simulink model "IEEE14_case"  (R2024b)
settings: Solver=FixedStepAuto  StartTime=0  StopTime=2  FixedStep=1e-7  RelTol=1e-3
values from neighbouring files (symbols this model uses):
  GFL_15_Bva = 0.009    [IEEE14_parameters.m]
  GFL_15_C_bus_pu = 7.179419    [IEEE14_parameters.m]
  GFL_15_f0 = 60    [IEEE14_parameters.m]
  GFL_15_I_id = 691.26967    [IEEE14_parameters.m]
  GFL_15_I_iq = 691.26967    [IEEE14_parameters.m]
  GFL_15_I_od = 45.2207    [IEEE14_parameters.m]
  GFL_15_I_oq = 45.2207    [IEEE14_parameters.m]
  GFL_15_I_pll = 0.78    [IEEE14_parameters.m]
  GFL_15_Kdi = 0.09    [IEEE14_parameters.m]
  GFL_15_Kdo = 0.9    [IEEE14_parameters.m]
  GFL_15_Kqi = 0.09    [IEEE14_parameters.m]
  GFL_15_Kqo = 0.9    [IEEE14_parameters.m]
  GFL_15_Lg_pu = 0.631447    [IEEE14_parameters.m]
  GFL_15_mode = 1    [IEEE14_parameters.m]
  GFL_15_P_id = 3.7166    [IEEE14_parameters.m]
  GFL_15_P_iq = 3.7166    [IEEE14_parameters.m]
  GFL_15_P_od = 0.4798    [IEEE14_parameters.m]
  GFL_15_P_oq = 0.4798    [IEEE14_parameters.m]
  GFL_15_P_pll = 290.42    [IEEE14_parameters.m]
  GFL_15_Qe_ref = 0.2    [IEEE14_parameters.m]
  GFL_15_Rg_pu = 0.024016    [IEEE14_parameters.m]
  GFL_15_Sbase = 1.000000e+4    (= 10000)    [IEEE14_parameters.m]
  GFL_15_Tdi = 0.01    [IEEE14_parameters.m]
  GFL_15_Tdo = 0.2    [IEEE14_parameters.m]
  GFL_15_Tqi = 0.01    [IEEE14_parameters.m]
  GFL_15_Tqo = 0.2    [IEEE14_parameters.m]
  GFL_15_Vbase = 380    [IEEE14_parameters.m]
  GFL_15_Vdc_ref = 1.011475    [IEEE14_parameters.m]
  GFL_15_Vdcbase = 700    [IEEE14_parameters.m]
  GFL_15_vq_ref = 0    [IEEE14_parameters.m]
  GFL_16_Bva = 0.002    [IEEE14_parameters.m]
  GFL_16_C_bus_pu = 7.179419    [IEEE14_parameters.m]
  GFL_16_f0 = 60    [IEEE14_parameters.m]
  GFL_16_I_id = 691.26967    [IEEE14_parameters.m]
  GFL_16_I_iq = 691.26967    [IEEE14_parameters.m]
  GFL_16_I_od = 45.2207    [IEEE14_parameters.m]
  GFL_16_I_oq = 45.2207    [IEEE14_parameters.m]
  GFL_16_I_pll = 0.78    [IEEE14_parameters.m]
  GFL_16_Kdi = 0.05    [IEEE14_parameters.m]
  GFL_16_Kdo = 0.5    [IEEE14_parameters.m]
  GFL_16_Kqi = 0.05    [IEEE14_parameters.m]
  GFL_16_Kqo = 0.5    [IEEE14_parameters.m]
  GFL_16_Lg_pu = 0.631447    [IEEE14_parameters.m]
  GFL_16_mode = 1    [IEEE14_parameters.m]
  GFL_16_P_id = 3.7166    [IEEE14_parameters.m]
  GFL_16_P_iq = 3.7166    [IEEE14_parameters.m]
  GFL_16_P_od = 0.4798    [IEEE14_parameters.m]
  GFL_16_P_oq = 0.4798    [IEEE14_parameters.m]
  GFL_16_P_pll = 290.42    [IEEE14_parameters.m]
  GFL_16_Qe_ref = 0.2    [IEEE14_parameters.m]
  GFL_16_Rg_pu = 0.024016    [IEEE14_parameters.m]
  GFL_16_Sbase = 1.000000e+4    (= 10000)    [IEEE14_parameters.m]
  GFL_16_Tdi = 0.01    [IEEE14_parameters.m]
  GFL_16_Tdo = 0.2    [IEEE14_parameters.m]
  GFL_16_Tqi = 0.01    [IEEE14_parameters.m]
  GFL_16_Tqo = 0.2    [IEEE14_parameters.m]
  GFL_16_Vbase = 380    [IEEE14_parameters.m]
  GFL_16_Vdc_ref = 1.01144    [IEEE14_parameters.m]
  GFL_16_Vdcbase = 700    [IEEE14_parameters.m]
  GFL_16_vq_ref = 0    [IEEE14_parameters.m]
  GFL_17_Bva = 0.002    [IEEE14_parameters.m]
  GFL_17_C_bus_pu = 7.179419    [IEEE14_parameters.m]
  GFL_17_f0 = 60    [IEEE14_parameters.m]
  GFL_17_I_id = 691.26967    [IEEE14_parameters.m]
  GFL_17_I_iq = 691.26967    [IEEE14_parameters.m]
  GFL_17_I_od = 45.2207    [IEEE14_parameters.m]
  GFL_17_I_oq = 45.2207    [IEEE14_parameters.m]
  GFL_17_I_pll = 0.78    [IEEE14_parameters.m]
  GFL_17_Kdi = 0.05    [IEEE14_parameters.m]
  GFL_17_Kdo = 0.5    [IEEE14_parameters.m]
  GFL_17_Kqi = 0.05    [IEEE14_parameters.m]
  GFL_17_Kqo = 0.5    [IEEE14_parameters.m]
  GFL_17_Lg_pu = 0.631447    [IEEE14_parameters.m]
  GFL_17_mode = 1    [IEEE14_parameters.m]
  GFL_17_P_id = 3.7166    [IEEE14_parameters.m]
  GFL_17_P_iq = 3.7166    [IEEE14_parameters.m]
  GFL_17_P_od = 0.4798    [IEEE14_parameters.m]
  GFL_17_P_oq = 0.4798    [IEEE14_parameters.m]
  GFL_17_P_pll = 290.42    [IEEE14_parameters.m]
  GFL_17_Qe_ref = 0.2    [IEEE14_parameters.m]
  GFL_17_Rg_pu = 0.024016    [IEEE14_parameters.m]
  GFL_17_Sbase = 1.000000e+4    (= 10000)    [IEEE14_parameters.m]
  GFL_17_Tdi = 0.01    [IEEE14_parameters.m]
  GFL_17_Tdo = 0.2    [IEEE14_parameters.m]
  GFL_17_Tqi = 0.01    [IEEE14_parameters.m]
  GFL_17_Tqo = 0.2    [IEEE14_parameters.m]
  GFL_17_Vbase = 380    [IEEE14_parameters.m]
  GFL_17_Vdc_ref = 1.011632    [IEEE14_parameters.m]
  GFL_17_Vdcbase = 700    [IEEE14_parameters.m]
  GFL_17_vq_ref = 0    [IEEE14_parameters.m]
  GFL_18_Bva = 0.002    [IEEE14_parameters.m]
  GFL_18_C_bus_pu = 7.179419    [IEEE14_parameters.m]
  GFL_18_f0 = 60    [IEEE14_parameters.m]
  GFL_18_I_id = 691.26967    [IEEE14_parameters.m]
  GFL_18_I_iq = 691.26967    [IEEE14_parameters.m]
  GFL_18_I_od = 45.2207    [IEEE14_parameters.m]
  GFL_18_I_oq = 45.2207    [IEEE14_parameters.m]
  GFL_18_I_pll = 0.78    [IEEE14_parameters.m]
  GFL_18_Kdi = 0.05    [IEEE14_parameters.m]
  GFL_18_Kdo = 0.5    [IEEE14_parameters.m]
  GFL_18_Kqi = 0.05    [IEEE14_parameters.m]
  GFL_18_Kqo = 0.5    [IEEE14_parameters.m]
  GFL_18_Lg_pu = 0.631447    [IEEE14_parameters.m]
  GFL_18_mode = 1    [IEEE14_parameters.m]
  GFL_18_P_id = 3.7166    [IEEE14_parameters.m]
  GFL_18_P_iq = 3.7166    [IEEE14_parameters.m]
  GFL_18_P_od = 0.4798    [IEEE14_parameters.m]
  GFL_18_P_oq = 0.4798    [IEEE14_parameters.m]
  GFL_18_P_pll = 290.42    [IEEE14_parameters.m]
  GFL_18_Qe_ref = 0.2    [IEEE14_parameters.m]
  GFL_18_Rg_pu = 0.024016    [IEEE14_parameters.m]
  GFL_18_Sbase = 1.000000e+4    (= 10000)    [IEEE14_parameters.m]
  GFL_18_Tdi = 0.01    [IEEE14_parameters.m]
  GFL_18_Tdo = 0.2    [IEEE14_parameters.m]
  GFL_18_Tqi = 0.01    [IEEE14_parameters.m]
  GFL_18_Tqo = 0.2    [IEEE14_parameters.m]
  GFL_18_Vbase = 380    [IEEE14_parameters.m]
  GFL_18_Vdc_ref = 1.011572    [IEEE14_parameters.m]
  GFL_18_Vdcbase = 700    [IEEE14_parameters.m]
  GFL_18_vq_ref = 0    [IEEE14_parameters.m]
  ... (+180 more)
(part 20 of 25)

== system IEEE14_case/SG_D_3/d_psi_fd_SG_D_3_block ==
  note: d_psi_fd_SG_D_3 in case14gfl
      | $-\frac{\psi _{\mathrm{fd},\mathrm{SG},D,3}-E_{\mathrm{fd},\mathrm{SG},D,3}+\left(x_{d}-x_{\mathrm{dd}}\right)\,\left(\frac{\frac{\psi _{\mathrm{1d},\mathrm{SG},D,3}\,\left(x_{\mathrm{dd}}-x_{\mathrm{ddd}}\right)}{x_{\mathrm{dd}}-x_{l}}-\psi _{d,\mathrm{SG},D,3}+\frac{\psi _{\mathrm{fd},\mathrm{SG},D,3}\,\left(x_{\mathrm{ddd}}-x_{l}\right)}{x_{\mathrm{dd}}-x_{l}}}{x_{\mathrm{ddd}}}-\frac{\left(x_{\mathrm{dd}}-x_{\mathrm{ddd}}\right)\,\left(\psi _{\mathrm{1d},\mathrm{SG},D,3}-\psi _{\mathrm{fd},\mathrm{SG},D,3}+\frac{\left(x_{\mathrm{dd}}-x_{l}\right)\,\left(\frac{\psi _{\mathrm{1d},\mathrm{SG},D,3}\,\left(x_{\mathrm{dd}}-x_{\mathrm{ddd}}\right)}{x_{\mathrm{dd}}-x_{l}}-\psi _{d,\mathrm{SG},D,3}+\frac{\psi _{\mathrm{fd},\mathrm{SG},D,3}\,\left(x_{\mathrm{ddd}}-x_{l}\right)}{x_{\mathrm{dd}}-x_{l}}\right)}{x_{\mathrm{ddd}}}\right)}{{\left(x_{\mathrm{dd}}-x_{l}\right)}^2}\right)}{T_{\mathrm{dd}}}$
      | Automatically generated on 2025-10-09 21:31:58 .
  State_E_fd_SG_D_3_d78e2 : Inport
  State_psi_fd_SG_D_3_1ca94 : Inport  Port=2
  State_psi_1d_SG_D_3_100d0 : Inport  Port=3
  State_psi_fd_SG_D_3_1fedc : Inport  Port=4
  State_psi_1d_SG_D_3_43bed : Inport  Port=5
  State_psi_d_SG_D_3_d3054 : Inport  Port=6
  State_psi_fd_SG_D_3_13cfd : Inport  Port=7
  State_psi_1d_SG_D_3_3ce6e : Inport  Port=8
  State_psi_d_SG_D_3_4847b : Inport  Port=9
  State_psi_fd_SG_D_3_01d8a : Inport  Port=10
  Add_80d2e : Sum
  Add_c54d7 : Sum
  Constant_-1_b236f : Constant  Value=-1
  Constant_-1_bec81 : Constant  Value=-1
  Constant_-1_d1f6f : Constant  Value=-1
  Constant_2.0_9c0bc : Constant  Value=2.0
  Constant_T_dd_bb507 : Constant  Value=T_dd
  Constant_x_d_3177e : Constant  Value=x_d
  Constant_x_dd_197e1 : Constant  Value=x_dd
  Constant_x_dd_2f9f2 : Constant  Value=x_dd
  Constant_x_dd_2fa42 : Constant  Value=x_dd
  Constant_x_dd_34495 : Constant  Value=x_dd
  Constant_x_dd_5dc80 : Constant  Value=x_dd
  Constant_x_dd_8bf3f : Constant  Value=x_dd
  Constant_x_dd_a9902 : Constant  Value=x_dd
  Constant_x_dd_c1224 : Constant  Value=x_dd
  Constant_x_dd_d2500 : Constant  Value=x_dd
  Constant_x_dd_f7ff0 : Constant  Value=x_dd
  Constant_x_ddd_238d1 : Constant  Value=x_ddd
  Constant_x_ddd_5390a : Constant  Value=x_ddd
  Constant_x_ddd_826ba : Constant  Value=x_ddd
  Constant_x_ddd_b0317 : Constant  Value=x_ddd
  Constant_x_ddd_b32cc : Constant  Value=x_ddd
  Constant_x_ddd_c2563 : Constant  Value=x_ddd
  Constant_x_ddd_db75c : Constant  Value=x_ddd
  Constant_x_l_1a217 : Constant  Value=x_l
  Constant_x_l_22cc2 : Constant  Value=x_l
  Constant_x_l_244ba : Constant  Value=x_l
  Constant_x_l_454cb : Constant  Value=x_l
  Constant_x_l_5313e : Constant  Value=x_l
  Constant_x_l_96c37 : Constant  Value=x_l
  Constant_x_l_de542 : Constant  Value=x_l
  Constant_x_l_e5b53 : Constant  Value=x_l
  Divide_0852c : Product  Inputs=*/
  Divide_3c28e : Product  Inputs=*/
  Divide_3c654 : Product  Inputs=*/
  Divide_63bfa : Product  Inputs=*/
  Divide_677e2 : Product  Inputs=*/
  Divide_9dd51 : Product  Inputs=*/
  Divide_a3d2d : Product  Inputs=*/
  Divide_c5de7 : Product  Inputs=*/
  Power_b9f7a : Math  Operator=pow
  Product_029d7 : Product
  Product_1e69a : Product
  Product_2ea94 : Product
  Product_9be52 : Product
  Product_a7353 : Product
  Product_b7520 : Product
  Product_b932f : Product
  Product_c4689 : Product
  Product_d1d0a : Product
  Product_dc8c2 : Product
  Subtract_0348b : Sum  Inputs=+-
  Subtract_12722 : Sum  Inputs=+-
  Subtract_267a6 : Sum  Inputs=+-
  Subtract_26a75 : Sum  Inputs=+-
  Subtract_468ee : Sum  Inputs=+-
  Subtract_48e53 : Sum  Inputs=+-
  Subtract_4fd9e : Sum  Inputs=+-
  Subtract_5d9ec : Sum  Inputs=+-
  Subtract_60539 : Sum  Inputs=+-
  Subtract_67c8f : Sum  Inputs=+-
  Subtract_905f1 : Sum  Inputs=+-
  Subtract_a0641 : Sum  Inputs=+-
  Subtract_a2941 : Sum  Inputs=+-
  Subtract_a6db3 : Sum  Inputs=+-
  Subtract_b8cef : Sum  Inputs=+-
  Subtract_c861a : Sum  Inputs=+-
  Subtract_db6b7 : Sum  Inputs=+-
  Subtract_ddf1e : Sum  Inputs=+-
  Subtract_df264 : Sum  Inputs=+-
  Blockout_d_psi_fd_SG_D_3_d4122 : Outport
  wires:
  Product_a7353/1 -> Divide_3c28e/1
  Constant_-1_b236f/1 -> Product_c4689/1
  Subtract_468ee/1 -> Product_2ea94/2
  State_psi_1d_SG_D_3_43bed/1 -> Product_c4689/2
  Constant_x_l_5313e/1 -> Subtract_a2941/2
  Constant_x_dd_5dc80/1 -> Subtract_468ee/1
  Constant_x_ddd_b32cc/1 -> Subtract_468ee/2
  Product_c4689/1 -> Product_2ea94/1
  Constant_x_dd_a9902/1 -> Subtract_db6b7/1
  Constant_x_l_454cb/1 -> Subtract_db6b7/2
  Constant_x_ddd_5390a/1 -> Subtract_5d9ec/2
  Constant_x_ddd_b0317/1 -> Subtract_26a75/1
  Constant_x_l_244ba/1 -> Subtract_26a75/2
  Product_b932f/1 -> Product_d1d0a/1
  Product_2ea94/1 -> Divide_3c654/1
  Subtract_db6b7/1 -> Divide_3c654/2
  State_psi_fd_SG_D_3_13cfd/1 -> Product_029d7/1
  Constant_x_ddd_db75c/1 -> Subtract_a2941/1
  Subtract_26a75/1 -> Product_029d7/2
  Constant_x_dd_8bf3f/1 -> Subtract_c861a/1
  Constant_-1_bec81/1 -> Product_b932f/1
  Constant_x_l_e5b53/1 -> Subtract_c861a/2
  Product_d1d0a/1 -> Divide_677e2/1
  Divide_3c654/1 -> Add_80d2e/1
  Product_b7520/1 -> Divide_0852c/1
  State_psi_d_SG_D_3_d3054/1 -> Add_80d2e/2
  State_psi_fd_SG_D_3_01d8a/1 -> Product_b7520/1
  Product_029d7/1 -> Divide_a3d2d/1
  Constant_x_dd_197e1/1 -> Subtract_905f1/1
  Subtract_c861a/1 -> Divide_a3d2d/2
  Constant_x_l_96c37/1 -> Subtract_ddf1e/2
  Constant_x_dd_d2500/1 -> Subtract_b8cef/1
  Subtract_267a6/1 -> Product_dc8c2/2
  Constant_x_l_1a217/1 -> Subtract_b8cef/2
  Divide_677e2/1 -> Add_c54d7/1
  Constant_x_ddd_826ba/1 -> Divide_3c28e/2
  Add_80d2e/1 -> Subtract_12722/1
  Divide_a3d2d/1 -> Subtract_12722/2
  State_psi_1d_SG_D_3_3ce6e/1 -> Product_b932f/2
  Constant_x_l_de542/1 -> Subtract_905f1/2
  Constant_x_dd_2f9f2/1 -> Subtract_5d9ec/1
  Subtract_b8cef/1 -> Product_a7353/1
  Add_c54d7/1 -> Subtract_67c8f/1
  Subtract_12722/1 -> Product_a7353/2
  Subtract_5d9ec/1 -> Product_d1d0a/2
  Constant_x_dd_f7ff0/1 -> Subtract_60539/1
  Constant_x_l_22cc2/1 -> Subtract_60539/2
  Subtract_a2941/1 -> Product_b7520/2
  Constant_x_dd_34495/1 -> Subtract_267a6/1
  Constant_x_ddd_238d1/1 -> Subtract_267a6/2
  Product_dc8c2/1 -> Product_9be52/1
  State_psi_1d_SG_D_3_100d0/1 -> Subtract_df264/1
  Subtract_60539/1 -> Divide_677e2/2
  State_psi_fd_SG_D_3_1fedc/1 -> Subtract_df264/2
  Constant_-1_d1f6f/1 -> Product_dc8c2/1
  Subtract_df264/1 -> Subtract_a0641/1
  Divide_3c28e/1 -> Subtract_a0641/2
  Constant_x_dd_c1224/1 -> Subtract_ddf1e/1
  Divide_0852c/1 -> Subtract_67c8f/2
  State_psi_d_SG_D_3_4847b/1 -> Add_c54d7/2
  Subtract_905f1/1 -> Divide_0852c/2
  Subtract_a0641/1 -> Product_9be52/2
  Subtract_ddf1e/1 -> Power_b9f7a/1
  Constant_2.0_9c0bc/1 -> Power_b9f7a/2
  Product_9be52/1 -> Divide_c5de7/1
  Subtract_48e53/1 -> Product_1e69a/2
  Power_b9f7a/1 -> Divide_c5de7/2
  Subtract_67c8f/1 -> Divide_63bfa/1
  Constant_x_ddd_c2563/1 -> Divide_63bfa/2
  Constant_x_d_3177e/1 -> Subtract_0348b/1
  Constant_x_dd_2fa42/1 -> Subtract_0348b/2
  Divide_c5de7/1 -> Subtract_48e53/1
  Divide_63bfa/1 -> Subtract_48e53/2
  State_E_fd_SG_D_3_d78e2/1 -> Subtract_a6db3/1
  State_psi_fd_SG_D_3_1ca94/1 -> Subtract_a6db3/2
  Subtract_0348b/1 -> Product_1e69a/1
  Subtract_a6db3/1 -> Subtract_4fd9e/1
  Product_1e69a/1 -> Subtract_4fd9e/2
  Subtract_4fd9e/1 -> Divide_9dd51/1
  Constant_T_dd_bb507/1 -> Divide_9dd51/2
  Divide_9dd51/1 -> Blockout_d_psi_fd_SG_D_3_d4122/1

== system IEEE14_case/SG_D_3/d_psi_gq_SG_D_3_block ==
  note: d_psi_gq_SG_D_3 in case14gfl
      | $-\frac{\psi _{\mathrm{gq},\mathrm{SG},D,3}+\left(x_{q}-x_{\mathrm{qd}}\right)\,\left(\frac{\psi _{q,\mathrm{SG},D,3}+\frac{\psi _{\mathrm{gq},\mathrm{SG},D,3}\,\left(x_{l}-x_{\mathrm{qdd}}\right)}{x_{l}-x_{\mathrm{qd}}}+\frac{\psi _{\mathrm{kq},\mathrm{SG},D,3}\,\left(x_{\mathrm{qd}}-x_{\mathrm{qdd}}\right)}{x_{l}-x_{\mathrm{qd}}}}{x_{\mathrm{qdd}}}+\frac{\left(x_{\mathrm{qd}}-x_{\mathrm{qdd}}\right)\,\left(\psi _{\mathrm{gq},\mathrm{SG},D,3}+\psi _{\mathrm{kq},\mathrm{SG},D,3}+\frac{\left(x_{l}-x_{\mathrm{qd}}\right)\,\left(\psi _{q,\mathrm{SG},D,3}+\frac{\psi _{\mathrm{gq},\mathrm{SG},D,3}\,\left(x_{l}-x_{\mathrm{qdd}}\right)}{x_{l}-x_{\mathrm{qd}}}+\frac{\psi _{\mathrm{kq},\mathrm{SG},D,3}\,\left(x_{\mathrm{qd}}-x_{\mathrm{qdd}}\right)}{x_{l}-x_{\mathrm{qd}}}\right)}{x_{\mathrm{qdd}}}\right)}{{\left(x_{l}-x_{\mathrm{qd}}\right)}^2}\right)}{T_{\mathrm{qd}}}$
      | Automatically generated on 2025-10-09 21:32:05 .
  State_psi_gq_SG_D_3_61d89 : Inport
  State_psi_gq_SG_D_3_d2fbb : Inport  Port=2
  State_psi_kq_SG_D_3_dfb0b : Inport  Port=3
  State_psi_gq_SG_D_3_45fb4 : Inport  Port=4
  State_psi_kq_SG_D_3_5ef0d : Inport  Port=5
  State_psi_q_SG_D_3_2ea70 : Inport  Port=6
  State_psi_gq_SG_D_3_a842f : Inport  Port=7
  State_psi_kq_SG_D_3_da800 : Inport  Port=8
  State_psi_q_SG_D_3_77fff : Inport  Port=9
  Add_74d59 : Sum
  Add_80cf5 : Sum
  Add_88f67 : Sum
  Add_8b6d3 : Sum
  Add_96fed : Sum
  Add_a22ad : Sum
  Add_a2434 : Sum
  Add_a3f81 : Sum
  Add_ba19f : Sum
  Add_e5f57 : Sum
  Add_f7575 : Sum
  Add_fd6a4 : Sum
  Constant_-1_073cf : Constant  Value=-1
  Constant_-1_20b8e : Constant  Value=-1
  Constant_-1_2bb06 : Constant  Value=-1
  Constant_-1_56ef8 : Constant  Value=-1
  Constant_-1_8bd02 : Constant  Value=-1
  Constant_-1_b65c8 : Constant  Value=-1
  Constant_-1_d4353 : Constant  Value=-1
  Constant_-1_de30b : Constant  Value=-1
  Constant_-1_e0e58 : Constant  Value=-1
  Constant_-1_e21ce : Constant  Value=-1
  Constant_2.0_954e6 : Constant  Value=2.0
  Constant_T_qd_c4423 : Constant  Value=T_qd
  Constant_x_l_1b9e5 : Constant  Value=x_l
  Constant_x_l_37ca8 : Constant  Value=x_l
  Constant_x_l_61450 : Constant  Value=x_l
  Constant_x_l_620cb : Constant  Value=x_l
  Constant_x_l_67d60 : Constant  Value=x_l
  Constant_x_l_adcf0 : Constant  Value=x_l
  Constant_x_l_bd098 : Constant  Value=x_l
  Constant_x_l_e870d : Constant  Value=x_l
  Constant_x_q_9ac0a : Constant  Value=x_q
  Constant_x_qd_04582 : Constant  Value=x_qd
  Constant_x_qd_08b35 : Constant  Value=x_qd
  Constant_x_qd_108e4 : Constant  Value=x_qd
  Constant_x_qd_11bce : Constant  Value=x_qd
  Constant_x_qd_321d1 : Constant  Value=x_qd
  Constant_x_qd_56097 : Constant  Value=x_qd
  Constant_x_qd_8aa9c : Constant  Value=x_qd
  Constant_x_qd_bf5b6 : Constant  Value=x_qd
  Constant_x_qd_d07df : Constant  Value=x_qd
  Constant_x_qd_f5adf : Constant  Value=x_qd
  Constant_x_qdd_27f87 : Constant  Value=x_qdd
  Constant_x_qdd_38975 : Constant  Value=x_qdd
  Constant_x_qdd_467dc : Constant  Value=x_qdd
  Constant_x_qdd_9fc2a : Constant  Value=x_qdd
  Constant_x_qdd_b0870 : Constant  Value=x_qdd
  Constant_x_qdd_b80c6 : Constant  Value=x_qdd
  Constant_x_qdd_f1e40 : Constant  Value=x_qdd
  Divide_00b90 : Product  Inputs=*/
  Divide_023dc : Product  Inputs=*/
  Divide_04f18 : Product  Inputs=*/
  Divide_3584c : Product  Inputs=*/
  Divide_4654a : Product  Inputs=*/
  Divide_4d5e7 : Product  Inputs=*/
  Divide_7f03c : Product  Inputs=*/
  Divide_b9d54 : Product  Inputs=*/
  Power_20cbb : Math  Operator=pow
  Product_0547a : Product
  Product_24422 : Product
  Product_2fb4f : Product
  Product_393f7 : Product
  Product_7f4c8 : Product
  Product_85de0 : Product
  Product_8b155 : Product
  Product_9510e : Product
  Product_a76f8 : Product
  Product_a7e86 : Product
  Product_b4629 : Product
  Product_b6ffa : Product
  Product_cb497 : Product
  Product_d015c : Product
  Product_de0ec : Product
  Product_e96c0 : Product
  Product_f73f6 : Product
  Subtract_0e44b : Sum  Inputs=+-
  Subtract_4270b : Sum  Inputs=+-
  Subtract_67b07 : Sum  Inputs=+-
  Subtract_96d88 : Sum  Inputs=+-
  Subtract_b3885 : Sum  Inputs=+-
  Subtract_c23cf : Sum  Inputs=+-
  Subtract_df751 : Sum  Inputs=+-
  Subtract_dfb85 : Sum  Inputs=+-
  Blockout_d_psi_gq_SG_D_3_d5302 : Outport
  wires:
  Constant_x_l_37ca8/1 -> Product_e96c0/2
  Constant_x_qd_108e4/1 -> Subtract_dfb85/1
  Add_e5f57/1 -> Product_b4629/1
  Constant_-1_2bb06/1 -> Product_0547a/1
  Add_fd6a4/1 -> Product_8b155/2
  Constant_x_qdd_b0870/1 -> Subtract_dfb85/2
  Constant_x_qd_04582/1 -> Add_e5f57/2
  Constant_x_l_adcf0/1 -> Product_0547a/2
  Constant_x_l_620cb/1 -> Product_9510e/2
  Add_ba19f/1 -> Divide_4654a/2
  State_psi_kq_SG_D_3_dfb0b/1 -> Add_a3f81/2
  Constant_x_qdd_9fc2a/1 -> Add_fd6a4/2
  Product_0547a/1 -> Add_fd6a4/1
  Constant_x_qd_bf5b6/1 -> Add_ba19f/2
  Product_393f7/1 -> Product_f73f6/1
  Constant_-1_e0e58/1 -> Product_2fb4f/1
  Constant_-1_8bd02/1 -> Product_9510e/1
  Constant_-1_073cf/1 -> Product_85de0/1
  Constant_x_l_61450/1 -> Product_85de0/2
  Constant_-1_e21ce/1 -> Product_393f7/1
  Constant_-1_b65c8/1 -> Product_24422/1
  State_psi_gq_SG_D_3_45fb4/1 -> Product_8b155/1
  Product_2fb4f/1 -> Add_a2434/1
  Product_9510e/1 -> Add_a22ad/1
  Product_7f4c8/1 -> Add_ba19f/1
  Constant_x_qd_08b35/1 -> Add_a22ad/2
  Constant_-1_56ef8/1 -> Product_a7e86/1
  State_psi_kq_SG_D_3_5ef0d/1 -> Product_b6ffa/1
  Subtract_dfb85/1 -> Product_b6ffa/2
  Product_85de0/1 -> Add_88f67/1
  Add_a2434/1 -> Product_d015c/2
  Add_a22ad/1 -> Divide_3584c/2
  Constant_x_qd_f5adf/1 -> Add_88f67/2
  Product_8b155/1 -> Divide_3584c/1
  Constant_T_qd_c4423/1 -> Divide_023dc/2
  Product_a7e86/1 -> Add_74d59/1
  Product_b6ffa/1 -> Divide_00b90/1
  Product_a76f8/1 -> Divide_4654a/1
  Add_88f67/1 -> Divide_00b90/2
  Constant_-1_d4353/1 -> Product_cb497/1
  Constant_x_qdd_467dc/1 -> Divide_b9d54/2
  Constant_x_l_e870d/1 -> Product_cb497/2
  Divide_3584c/1 -> Subtract_df751/1
  Constant_x_qd_d07df/1 -> Subtract_c23cf/2
  Add_74d59/1 -> Divide_4d5e7/2
  Divide_00b90/1 -> Subtract_df751/2
  Constant_x_l_1b9e5/1 -> Product_2fb4f/2
  Product_cb497/1 -> Add_e5f57/1
  Constant_-1_de30b/1 -> Product_e96c0/1
  Constant_x_l_67d60/1 -> Product_a7e86/2
  Subtract_df751/1 -> Add_96fed/1
  State_psi_q_SG_D_3_2ea70/1 -> Add_96fed/2
  Constant_-1_20b8e/1 -> Product_7f4c8/1
  Constant_x_qdd_b80c6/1 -> Add_a2434/2
  Constant_x_qd_56097/1 -> Subtract_96d88/1
  Constant_x_qdd_38975/1 -> Subtract_96d88/2
  Constant_x_l_bd098/1 -> Product_7f4c8/2
  Add_96fed/1 -> Product_b4629/2
  Constant_x_qdd_27f87/1 -> Subtract_67b07/2
  State_psi_gq_SG_D_3_a842f/1 -> Product_d015c/1
  Constant_x_qd_8aa9c/1 -> Add_74d59/2
  Divide_7f03c/1 -> Subtract_b3885/1
  State_psi_kq_SG_D_3_da800/1 -> Product_a76f8/1
  Subtract_96d88/1 -> Product_a76f8/2
  Constant_x_qd_11bce/1 -> Subtract_67b07/1
  State_psi_gq_SG_D_3_d2fbb/1 -> Add_a3f81/1
  Product_b4629/1 -> Divide_b9d54/1
  Product_d015c/1 -> Divide_4d5e7/1
  Subtract_67b07/1 -> Product_393f7/2
  Add_a3f81/1 -> Subtract_0e44b/1
  Divide_b9d54/1 -> Subtract_0e44b/2
  Product_e96c0/1 -> Add_80cf5/1
  Constant_x_qd_321d1/1 -> Add_80cf5/2
  Divide_4d5e7/1 -> Subtract_4270b/1
  Divide_4654a/1 -> Subtract_4270b/2
  Subtract_0e44b/1 -> Product_f73f6/2
  Add_80cf5/1 -> Power_20cbb/1
  Constant_2.0_954e6/1 -> Power_20cbb/2
  Subtract_4270b/1 -> Add_f7575/1
  State_psi_q_SG_D_3_77fff/1 -> Add_f7575/2
  Product_f73f6/1 -> Divide_7f03c/1
  Power_20cbb/1 -> Divide_7f03c/2
  Add_f7575/1 -> Divide_04f18/1
  Constant_x_qdd_f1e40/1 -> Divide_04f18/2
  Constant_x_q_9ac0a/1 -> Subtract_c23cf/1
  Divide_04f18/1 -> Subtract_b3885/2
  State_psi_gq_SG_D_3_61d89/1 -> Product_24422/2
  Subtract_c23cf/1 -> Product_de0ec/1
  Subtract_b3885/1 -> Product_de0ec/2
  Product_24422/1 -> Add_8b6d3/1
  Product_de0ec/1 -> Add_8b6d3/2
  Add_8b6d3/1 -> Divide_023dc/1
  Divide_023dc/1 -> Blockout_d_psi_gq_SG_D_3_d5302/1

== system IEEE14_case/SG_D_3/d_psi_kq_SG_D_3_block ==
  note: d_psi_kq_SG_D_3 in case14gfl
      | $-\frac{\psi _{\mathrm{gq},\mathrm{SG},D,3}+\psi _{\mathrm{kq},\mathrm{SG},D,3}+\frac{\left(x_{l}-x_{\mathrm{qd}}\right)\,\left(\psi _{q,\mathrm{SG},D,3}+\frac{\psi _{\mathrm{gq},\mathrm{SG},D,3}\,\left(x_{l}-x_{\mathrm{qdd}}\right)}{x_{l}-x_{\mathrm{qd}}}+\frac{\psi _{\mathrm{kq},\mathrm{SG},D,3}\,\left(x_{\mathrm{qd}}-x_{\mathrm{qdd}}\right)}{x_{l}-x_{\mathrm{qd}}}\right)}{x_{\mathrm{qdd}}}}{T_{\mathrm{qdd}}}$
      | Automatically generated on 2025-10-09 21:32:08 .
  State_psi_gq_SG_D_3_5f103 : Inport
  State_psi_kq_SG_D_3_66cec : Inport  Port=2
  State_psi_gq_SG_D_3_d768f : Inport  Port=3
  State_psi_kq_SG_D_3_3bd28 : Inport  Port=4
  State_psi_q_SG_D_3_41969 : Inport  Port=5
  Add_0ddbf : Sum
  Add_1aa52 : Sum
  Add_51ab7 : Sum
  Add_8654d : Sum
  Add_a36c4 : Sum
  Add_d72a9 : Sum
  Constant_-1_02b02 : Constant  Value=-1
  Constant_-1_0d781 : Constant  Value=-1
  Constant_-1_99886 : Constant  Value=-1
  Constant_-1_d75ef : Constant  Value=-1
  Constant_-1_d97d4 : Constant  Value=-1
  Constant_T_qdd_6762e : Constant  Value=T_qdd
  Constant_x_l_0960a : Constant  Value=x_l
  Constant_x_l_772c1 : Constant  Value=x_l
  Constant_x_l_c951c : Constant  Value=x_l
  Constant_x_l_f41cc : Constant  Value=x_l
  Constant_x_qd_7ea52 : Constant  Value=x_qd
  Constant_x_qd_b6964 : Constant  Value=x_qd
  Constant_x_qd_c158b : Constant  Value=x_qd
  Constant_x_qd_d1d5f : Constant  Value=x_qd
  Constant_x_qdd_3258c : Constant  Value=x_qdd
  Constant_x_qdd_6ba2b : Constant  Value=x_qdd
  Constant_x_qdd_72f52 : Constant  Value=x_qdd
  Divide_28285 : Product  Inputs=*/
  Divide_2d6a6 : Product  Inputs=*/
  Divide_38392 : Product  Inputs=*/
  Divide_ec21f : Product  Inputs=*/
  Product_064ec : Product
  Product_0c2ce : Product
  Product_5b1b5 : Product
  Product_67d15 : Product
  Product_7b1df : Product
  Product_8a972 : Product
  Product_de990 : Product
  Product_ed944 : Product
  Subtract_516d0 : Sum  Inputs=+-
  Subtract_808b2 : Sum  Inputs=+-
  Subtract_a4f43 : Sum  Inputs=+-
  Blockout_d_psi_kq_SG_D_3_bc348 : Outport
  wires:
  State_psi_q_SG_D_3_41969/1 -> Add_1aa52/2
  Constant_-1_d75ef/1 -> Product_0c2ce/1
  Constant_-1_99886/1 -> Product_de990/1
  Constant_-1_0d781/1 -> Product_ed944/1
  Constant_x_l_0960a/1 -> Product_0c2ce/2
  Constant_x_qdd_72f52/1 -> Add_51ab7/2
  Product_8a972/1 -> Add_8654d/1
  Constant_x_l_772c1/1 -> Product_de990/2
  Constant_x_qd_c158b/1 -> Subtract_516d0/1
  Product_de990/1 -> Add_51ab7/1
  Constant_x_l_c951c/1 -> Product_5b1b5/2
  Constant_x_qdd_6ba2b/1 -> Subtract_516d0/2
  Constant_-1_d97d4/1 -> Product_8a972/1
  Constant_x_l_f41cc/1 -> Product_8a972/2
  State_psi_gq_SG_D_3_d768f/1 -> Product_67d15/1
  Add_51ab7/1 -> Product_67d15/2
  Add_1aa52/1 -> Product_7b1df/2
  Product_0c2ce/1 -> Add_d72a9/1
  Constant_x_qd_d1d5f/1 -> Add_d72a9/2
  State_psi_kq_SG_D_3_3bd28/1 -> Product_064ec/1
  Subtract_516d0/1 -> Product_064ec/2
  Add_d72a9/1 -> Divide_2d6a6/2
  Constant_x_qd_b6964/1 -> Add_8654d/2
  Product_67d15/1 -> Divide_2d6a6/1
  Product_064ec/1 -> Divide_ec21f/1
  Add_8654d/1 -> Divide_ec21f/2
  Constant_-1_02b02/1 -> Product_5b1b5/1
  Divide_2d6a6/1 -> Subtract_a4f43/1
  Add_a36c4/1 -> Divide_38392/1
  Divide_ec21f/1 -> Subtract_a4f43/2
  Divide_38392/1 -> Blockout_d_psi_kq_SG_D_3_bc348/1
  Product_5b1b5/1 -> Add_0ddbf/1
  Constant_x_qd_7ea52/1 -> Add_0ddbf/2
  Subtract_a4f43/1 -> Add_1aa52/1
  State_psi_gq_SG_D_3_5f103/1 -> Product_ed944/2
  Add_0ddbf/1 -> Product_7b1df/1
  Constant_T_qdd_6762e/1 -> Divide_38392/2
  Product_ed944/1 -> Subtract_808b2/1
  State_psi_kq_SG_D_3_66cec/1 -> Subtract_808b2/2
  Product_7b1df/1 -> Divide_28285/1
  Constant_x_qdd_3258c/1 -> Divide_28285/2
  Subtract_808b2/1 -> Add_a36c4/1
  Divide_28285/1 -> Add_a36c4/2

== system IEEE14_case/SG_D_3/d_psi_q_SG_D_3_block ==
  note: d_psi_q_SG_D_3 in case14gfl
      | $2\,\pi \,f_{0}\,\left(v_{d,\mathrm{SG},D,3}\,\cos\left(\theta _{\mathrm{SG},D,3}\right)+v_{q,\mathrm{SG},D,3}\,\sin\left(\theta _{\mathrm{SG},D,3}\right)-\frac{R_{a}\,\left(\psi _{q,\mathrm{SG},D,3}+\frac{\psi _{\mathrm{gq},\mathrm{SG},D,3}\,\left(x_{l}-x_{\mathrm{qdd}}\right)}{x_{l}-x_{\mathrm{qd}}}+\frac{\psi _{\mathrm{kq},\mathrm{SG},D,3}\,\left(x_{\mathrm{qd}}-x_{\mathrm{qdd}}\right)}{x_{l}-x_{\mathrm{qd}}}\right)}{x_{\mathrm{qdd}}}-\frac{\psi _{d,\mathrm{SG},D,3}\,w_{\mathrm{SG},D,3}}{2\,f_{0}\,\pi }\right)$
      | Automatically generated on 2025-10-09 21:31:53 .
  State_psi_gq_SG_D_3_7cee6 : Inport
  State_psi_kq_SG_D_3_9869f : Inport  Port=2
  State_psi_q_SG_D_3_e7c3e : Inport  Port=3
  Input_v_d_SG_D_3_62f18 : Inport  Port=4
  State_theta_SG_D_3_1d26c : Inport  Port=5
  Input_v_q_SG_D_3_5442f : Inport  Port=6
  State_theta_SG_D_3_b7f72 : Inport  Port=7
  State_psi_d_SG_D_3_6630b : Inport  Port=8
  State_w_SG_D_3_3bc6e : Inport  Port=9
  Add_4d8c9 : Sum
  Add_675a4 : Sum
  Add_9e2fe : Sum
  Add_a4c92 : Sum
  Add_e3814 : Sum
  Constant_-1_39a82 : Constant  Value=-1
  Constant_-1_3d702 : Constant  Value=-1
  Constant_-1_ad050 : Constant  Value=-1
  Constant_-2.0_6883f : Constant  Value=-2.0
  Constant_2.0_a20c9 : Constant  Value=2.0
  Constant_R_a_db5ad : Constant  Value=R_a
  Constant_f0_1ca5a : Constant  Value=f0
  Constant_f0_f3ce1 : Constant  Value=f0
  Constant_pi_13977 : Constant  Value=pi
  Constant_pi_1433e : Constant  Value=pi
  Constant_x_l_01e14 : Constant  Value=x_l
  Constant_x_l_16530 : Constant  Value=x_l
  Constant_x_l_48893 : Constant  Value=x_l
  Constant_x_qd_07b31 : Constant  Value=x_qd
  Constant_x_qd_c497d : Constant  Value=x_qd
  Constant_x_qd_c5bec : Constant  Value=x_qd
  Constant_x_qdd_37bb0 : Constant  Value=x_qdd
  Constant_x_qdd_c88d9 : Constant  Value=x_qdd
  Constant_x_qdd_d03d5 : Constant  Value=x_qdd
  Divide_24ee4 : Product  Inputs=*/
  Divide_4b10a : Product  Inputs=*/
  Divide_6ea3c : Product  Inputs=*/
  Divide_a49c9 : Product  Inputs=*/
  MathFunc_cos_273fa : Trigonometry  Operator=cos
  MathFunc_sin_0567a : Trigonometry
  Product_098df : Product
  Product_35f62 : Product
  Product_41dc2 : Product
  Product_695bc : Product
  Product_6a837 : Product
  Product_6dd1f : Product
  Product_759d2 : Product
  Product_9d5cc : Product
  Product_c2ec5 : Product
  Product_d4b9e : Product
  Product_dc931 : Product
  Product_dd8d8 : Product
  Product_ea9a3 : Product
  Product_fa1b1 : Product
  Subtract_0065d : Sum  Inputs=+-
  Subtract_5b699 : Sum  Inputs=+-
  Subtract_a39ab : Sum  Inputs=+-
  Subtract_b1ac8 : Sum  Inputs=+-
  Blockout_d_psi_q_SG_D_3_309b6 : Outport
  wires:
  Constant_x_qd_c497d/1 -> Subtract_a39ab/1
  Constant_pi_13977/1 -> Product_c2ec5/2
  Product_fa1b1/1 -> Divide_4b10a/1
  Constant_x_l_48893/1 -> Product_098df/2
  Constant_f0_1ca5a/1 -> Product_695bc/2
  State_w_SG_D_3_3bc6e/1 -> Product_ea9a3/2
  Constant_-1_ad050/1 -> Product_dd8d8/1
  Constant_x_qdd_37bb0/1 -> Add_a4c92/2
  Input_v_d_SG_D_3_62f18/1 -> Product_35f62/1
  Constant_x_qdd_d03d5/1 -> Subtract_a39ab/2
  Constant_x_l_16530/1 -> Product_dd8d8/2
  Divide_24ee4/1 -> Add_675a4/2
  Product_dd8d8/1 -> Add_a4c92/1
  Constant_2.0_a20c9/1 -> Product_c2ec5/1
  Add_e3814/1 -> Product_fa1b1/2
  Constant_-1_3d702/1 -> Product_098df/1
  Constant_x_qd_07b31/1 -> Add_9e2fe/2
  Constant_-1_39a82/1 -> Product_41dc2/1
  Subtract_5b699/1 -> Subtract_b1ac8/1
  Constant_x_l_01e14/1 -> Product_41dc2/2
  Subtract_b1ac8/1 -> Add_675a4/1
  Constant_f0_f3ce1/1 -> Product_6a837/2
  State_theta_SG_D_3_b7f72/1 -> MathFunc_sin_0567a/1
  Constant_x_qd_c5bec/1 -> Add_4d8c9/2
  State_psi_gq_SG_D_3_7cee6/1 -> Product_759d2/1
  Add_a4c92/1 -> Product_759d2/2
  Product_c2ec5/1 -> Product_6a837/1
  Product_098df/1 -> Add_4d8c9/1
  State_psi_kq_SG_D_3_9869f/1 -> Product_9d5cc/1
  Subtract_a39ab/1 -> Product_9d5cc/2
  Product_41dc2/1 -> Add_9e2fe/1
  MathFunc_sin_0567a/1 -> Product_6dd1f/2
  Product_759d2/1 -> Divide_a49c9/1
  Product_6a837/1 -> Divide_24ee4/2
  Add_4d8c9/1 -> Divide_a49c9/2
  Product_9d5cc/1 -> Divide_6ea3c/1
  Add_9e2fe/1 -> Divide_6ea3c/2
  Input_v_q_SG_D_3_5442f/1 -> Product_6dd1f/1
  Divide_a49c9/1 -> Subtract_0065d/1
  Subtract_0065d/1 -> Add_e3814/1
  Divide_6ea3c/1 -> Subtract_0065d/2
  Divide_4b10a/1 -> Subtract_5b699/1
  State_psi_q_SG_D_3_e7c3e/1 -> Add_e3814/2
  Product_6dd1f/1 -> Subtract_b1ac8/2
  Constant_R_a_db5ad/1 -> Product_fa1b1/1
  State_theta_SG_D_3_1d26c/1 -> MathFunc_cos_273fa/1
  Constant_x_qdd_c88d9/1 -> Divide_4b10a/2
  MathFunc_cos_273fa/1 -> Product_35f62/2
  Constant_-2.0_6883f/1 -> Product_dc931/1
  Product_35f62/1 -> Subtract_5b699/2
  State_psi_d_SG_D_3_6630b/1 -> Product_ea9a3/1
  Constant_pi_1433e/1 -> Product_dc931/2
  Product_ea9a3/1 -> Divide_24ee4/1
  Product_dc931/1 -> Product_695bc/1
  Product_695bc/1 -> Product_d4b9e/1
  Add_675a4/1 -> Product_d4b9e/2
  Product_d4b9e/1 -> Blockout_d_psi_q_SG_D_3_309b6/1

== system IEEE14_case/SG_D_3/d_theta_SG_D_3_block ==
  note: d_theta_SG_D_3 in case14gfl
      | $w_{\mathrm{SG},D,3}-2\,\pi \,f_{0}$
      | Automatically generated on 2025-10-09 21:32:14 .
  State_w_SG_D_3_b92e8 : Inport
  Add_6e354 : Sum
  Constant_-2.0_89cfc : Constant  Value=-2.0
  Constant_f0_64c7c : Constant  Value=f0
  Constant_pi_da10d : Constant  Value=pi
  Product_6bf2a : Product
  Product_eca5a : Product
  Blockout_d_theta_SG_D_3_c1b15 : Outport
  wires:
  Constant_-2.0_89cfc/1 -> Product_6bf2a/1
  Constant_pi_da10d/1 -> Product_6bf2a/2
  State_w_SG_D_3_b92e8/1 -> Add_6e354/2
  Product_6bf2a/1 -> Product_eca5a/1
  Constant_f0_64c7c/1 -> Product_eca5a/2
  Product_eca5a/1 -> Add_6e354/1
  Add_6e354/1 -> Blockout_d_theta_SG_D_3_c1b15/1

== system IEEE14_case/SG_D_3/d_w_SG_D_3_block ==
  note: d_w_SG_D_3 in case14gfl
      | $\frac{2\,\pi \,T_{m,\mathrm{SG},D,3}\,f_{0}-D\,\left(w_{\mathrm{SG},D,3}-2\,\pi \,f_{0}\right)+2\,\pi \,f_{0}\,\left(\frac{\psi _{d,\mathrm{SG},D,3}\,\left(\psi _{q,\mathrm{SG},D,3}+\frac{\psi _{\mathrm{gq},\mathrm{SG},D,3}\,\left(x_{l}-x_{\mathrm{qdd}}\right)}{x_{l}-x_{\mathrm{qd}}}+\frac{\psi _{\mathrm{kq},\mathrm{SG},D,3}\,\left(x_{\mathrm{qd}}-x_{\mathrm{qdd}}\right)}{x_{l}-x_{\mathrm{qd}}}\right)}{x_{\mathrm{qdd}}}+\frac{\psi _{q,\mathrm{SG},D,3}\,\left(\frac{\psi _{\mathrm{1d},\mathrm{SG},D,3}\,\left(x_{\mathrm{dd}}-x_{\mathrm{ddd}}\right)}{x_{\mathrm{dd}}-x_{l}}-\psi _{d,\mathrm{SG},D,3}+\frac{\psi _{\mathrm{fd},\mathrm{SG},D,3}\,\left(x_{\mathrm{ddd}}-x_{l}\right)}{x_{\mathrm{dd}}-x_{l}}\right)}{x_{\mathrm{ddd}}}\right)}{2\,H}$
      | Automatically generated on 2025-10-09 21:32:13 .
  State_w_SG_D_3_2376b : Inport
  State_T_m_SG_D_3_41b09 : Inport  Port=2
  State_psi_d_SG_D_3_bb520 : Inport  Port=3
  State_psi_gq_SG_D_3_2aa1e : Inport  Port=4
  State_psi_kq_SG_D_3_d40a5 : Inport  Port=5
  State_psi_q_SG_D_3_648aa : Inport  Port=6
  State_psi_q_SG_D_3_f6aa0 : Inport  Port=7
  State_psi_1d_SG_D_3_c9bae : Inport  Port=8
  State_psi_d_SG_D_3_02a5f : Inport  Port=9
  State_psi_fd_SG_D_3_2ef0f : Inport  Port=10
  Add_194db : Sum
  Add_21348 : Sum
  Add_386c0 : Sum
  Add_5085e : Sum
  Add_57efb : Sum
  Add_60b79 : Sum
  Add_dc0bb : Sum
  Add_e89be : Sum
  Constant_-1_4fcdb : Constant  Value=-1
  Constant_-1_8a714 : Constant  Value=-1
  Constant_-1_9a439 : Constant  Value=-1
  Constant_-1_b336f : Constant  Value=-1
  Constant_-1_d614b : Constant  Value=-1
  Constant_-1_e8ddd : Constant  Value=-1
  Constant_-2.0_d37a3 : Constant  Value=-2.0
  Constant_2.0_13da0 : Constant  Value=2.0
  Constant_2.0_751c3 : Constant  Value=2.0
  Constant_2.0_d6ce2 : Constant  Value=2.0
  Constant_D_fcce1 : Constant  Value=D
  Constant_H_cb47e : Constant  Value=H
  Constant_f0_4be39 : Constant  Value=f0
  Constant_f0_b92a2 : Constant  Value=f0
  Constant_f0_ed958 : Constant  Value=f0
  Constant_pi_795c3 : Constant  Value=pi
  Constant_pi_80d89 : Constant  Value=pi
  Constant_pi_c7737 : Constant  Value=pi
  Constant_x_dd_76ae7 : Constant  Value=x_dd
  Constant_x_dd_9c992 : Constant  Value=x_dd
  Constant_x_dd_d9565 : Constant  Value=x_dd
  Constant_x_ddd_16ead : Constant  Value=x_ddd
  Constant_x_ddd_285e1 : Constant  Value=x_ddd
  Constant_x_ddd_7a6df : Constant  Value=x_ddd
  Constant_x_l_04285 : Constant  Value=x_l
  Constant_x_l_2bd50 : Constant  Value=x_l
  Constant_x_l_6486b : Constant  Value=x_l
  Constant_x_l_9f744 : Constant  Value=x_l
  Constant_x_l_a4b6d : Constant  Value=x_l
  Constant_x_l_c9de8 : Constant  Value=x_l
  Constant_x_qd_b3b3a : Constant  Value=x_qd
  Constant_x_qd_c2062 : Constant  Value=x_qd
  Constant_x_qd_d96ba : Constant  Value=x_qd
  Constant_x_qdd_616ff : Constant  Value=x_qdd
  Constant_x_qdd_8dcb2 : Constant  Value=x_qdd
  Constant_x_qdd_bc462 : Constant  Value=x_qdd
  Divide_1a8aa : Product  Inputs=*/
  Divide_1f673 : Product  Inputs=*/
  Divide_371c7 : Product  Inputs=*/
  Divide_8e73e : Product  Inputs=*/
  Divide_a6fb6 : Product  Inputs=*/
  Divide_c747d : Product  Inputs=*/
  Divide_efe9d : Product  Inputs=*/
  Product_1078e : Product
  Product_1f94c : Product
  Product_2426d : Product
  Product_2e846 : Product
  Product_3304d : Product
  Product_34e80 : Product
  Product_62a0c : Product
  Product_66535 : Product
  Product_66727 : Product
  Product_73b0f : Product
  Product_73f53 : Product
  Product_792c2 : Product
  Product_7bb8b : Product
  Product_837a9 : Product
  Product_87b9f : Product
  Product_88505 : Product
  Product_a045e : Product
  Product_a15ce : Product
  Product_a8813 : Product
  Product_aae2b : Product
  Product_e4866 : Product
  Product_f4ad8 : Product
  Subtract_0c780 : Sum  Inputs=+-
  Subtract_63de8 : Sum  Inputs=+-
  Subtract_8540f : Sum  Inputs=+-
  Subtract_86a9a : Sum  Inputs=+-
  Subtract_94680 : Sum  Inputs=+-
  Subtract_b470c : Sum  Inputs=+-
  Subtract_f97c0 : Sum  Inputs=+-
  Subtract_fef0a : Sum  Inputs=+-
  Blockout_d_w_SG_D_3_aa189 : Outport
  wires:
  Constant_x_qd_b3b3a/1 -> Subtract_94680/1
  Subtract_b470c/1 -> Product_a045e/2
  Subtract_fef0a/1 -> Divide_371c7/1
  Constant_-1_d614b/1 -> Product_66535/1
  Add_57efb/1 -> Product_88505/2
  Constant_x_qdd_bc462/1 -> Subtract_94680/2
  Subtract_63de8/1 -> Product_34e80/2
  Constant_x_l_04285/1 -> Product_66535/2
  State_psi_d_SG_D_3_02a5f/1 -> Add_21348/2
  Add_5085e/1 -> Divide_a6fb6/2
  Constant_x_dd_76ae7/1 -> Subtract_f97c0/1
  Constant_x_l_a4b6d/1 -> Product_66727/2
  Constant_-1_8a714/1 -> Product_837a9/1
  Divide_8e73e/1 -> Subtract_0c780/2
  Constant_x_ddd_7a6df/1 -> Subtract_b470c/2
  Constant_x_qdd_616ff/1 -> Add_57efb/2
  Constant_pi_795c3/1 -> Product_f4ad8/2
  Product_66535/1 -> Add_57efb/1
  Constant_-2.0_d37a3/1 -> Product_aae2b/1
  Constant_-1_b336f/1 -> Product_66727/1
  Constant_2.0_13da0/1 -> Product_73b0f/1
  Product_aae2b/1 -> Product_7bb8b/1
  Constant_-1_9a439/1 -> Product_3304d/1
  Subtract_86a9a/1 -> Add_194db/1
  Constant_x_l_6486b/1 -> Product_3304d/2
  Constant_x_l_c9de8/1 -> Subtract_63de8/2
  Constant_-1_e8ddd/1 -> Product_1f94c/1
  State_psi_1d_SG_D_3_c9bae/1 -> Product_1f94c/2
  Constant_x_dd_9c992/1 -> Subtract_b470c/1
  Product_1f94c/1 -> Product_a045e/1
  State_psi_gq_SG_D_3_2aa1e/1 -> Product_88505/1
  Constant_x_qd_d96ba/1 -> Add_5085e/2
  Product_66727/1 -> Add_5085e/1
  State_psi_kq_SG_D_3_d40a5/1 -> Product_a15ce/1
  Subtract_94680/1 -> Product_a15ce/2
  Product_73b0f/1 -> Product_a8813/1
  Product_7bb8b/1 -> Add_dc0bb/1
  Product_3304d/1 -> Add_386c0/1
  State_psi_q_SG_D_3_f6aa0/1 -> Product_792c2/1
  Constant_x_qd_c2062/1 -> Add_386c0/2
  Constant_x_l_9f744/1 -> Subtract_f97c0/2
  Constant_x_ddd_285e1/1 -> Subtract_63de8/1
  Constant_x_l_2bd50/1 -> Subtract_8540f/2
  Product_88505/1 -> Divide_a6fb6/1
  Product_a15ce/1 -> Divide_c747d/1
  Add_386c0/1 -> Divide_c747d/2
  Product_a045e/1 -> Divide_1f673/1
  Subtract_f97c0/1 -> Divide_1f673/2
  Constant_2.0_d6ce2/1 -> Product_f4ad8/1
  State_psi_fd_SG_D_3_2ef0f/1 -> Product_34e80/1
  Constant_x_dd_d9565/1 -> Subtract_8540f/1
  Divide_a6fb6/1 -> Subtract_86a9a/1
  Product_34e80/1 -> Divide_8e73e/1
  Divide_c747d/1 -> Subtract_86a9a/2
  Divide_1f673/1 -> Add_21348/1
  Product_87b9f/1 -> Subtract_fef0a/2
  Subtract_8540f/1 -> Divide_8e73e/2
  Constant_pi_80d89/1 -> Product_aae2b/2
  Constant_pi_c7737/1 -> Product_73b0f/2
  Constant_-1_4fcdb/1 -> Product_62a0c/1
  State_psi_d_SG_D_3_bb520/1 -> Product_62a0c/2
  State_psi_q_SG_D_3_648aa/1 -> Add_194db/2
  Add_21348/1 -> Subtract_0c780/1
  Constant_f0_b92a2/1 -> Product_7bb8b/2
  Product_62a0c/1 -> Product_2426d/1
  Add_194db/1 -> Product_2426d/2
  Subtract_0c780/1 -> Product_792c2/2
  Constant_D_fcce1/1 -> Product_837a9/2
  State_w_SG_D_3_2376b/1 -> Add_dc0bb/2
  Product_f4ad8/1 -> Product_73f53/1
  State_T_m_SG_D_3_41b09/1 -> Product_73f53/2
  Product_2426d/1 -> Divide_efe9d/1
  Constant_x_qdd_8dcb2/1 -> Divide_efe9d/2
  Product_792c2/1 -> Divide_1a8aa/1
  Constant_x_ddd_16ead/1 -> Divide_1a8aa/2
  Product_837a9/1 -> Product_e4866/1
  Add_dc0bb/1 -> Product_e4866/2
  Product_73f53/1 -> Product_2e846/1
  Constant_f0_4be39/1 -> Product_2e846/2
  Constant_f0_ed958/1 -> Product_a8813/2
  Divide_efe9d/1 -> Add_60b79/1
  Divide_1a8aa/1 -> Add_60b79/2
  Product_e4866/1 -> Add_e89be/1
  Product_2e846/1 -> Add_e89be/2
  Product_a8813/1 -> Product_87b9f/1
  Add_60b79/1 -> Product_87b9f/2
  Add_e89be/1 -> Subtract_fef0a/1
  Constant_2.0_751c3/1 -> Product_1078e/1
  Constant_H_cb47e/1 -> Product_1078e/2
  Product_1078e/1 -> Divide_371c7/2
  Divide_371c7/1 -> Blockout_d_w_SG_D_3_aa189/1

== system IEEE14_case/SG_D_3/i_d_SG_D_3_block ==
  note: i_d_SG_D_3 in case14gfl
      | $\frac{\sin\left(\theta _{\mathrm{SG},D,3}\right)\,\left(\frac{\psi _{\mathrm{1d},\mathrm{SG},D,3}\,\left(x_{\mathrm{dd}}-x_{\mathrm{ddd}}\right)}{x_{\mathrm{dd}}-x_{l}}-\psi _{d,\mathrm{SG},D,3}+\frac{\psi _{\mathrm{fd},\mathrm{SG},D,3}\,\left(x_{\mathrm{ddd}}-x_{l}\right)}{x_{\mathrm{dd}}-x_{l}}\right)}{x_{\mathrm{ddd}}}-\frac{\cos\left(\theta _{\mathrm{SG},D,3}\right)\,\left(\psi _{q,\mathrm{SG},D,3}+\frac{\psi _{\mathrm{gq},\mathrm{SG},D,3}\,\left(x_{l}-x_{\mathrm{qdd}}\right)}{x_{l}-x_{\mathrm{qd}}}+\frac{\psi _{\mathrm{kq},\mathrm{SG},D,3}\,\left(x_{\mathrm{qd}}-x_{\mathrm{qdd}}\right)}{x_{l}-x_{\mathrm{qd}}}\right)}{x_{\mathrm{qdd}}}$
      | Automatically generated on 2025-10-09 21:32:32 .
  State_psi_gq_SG_D_3_ef59b : Inport
  State_psi_kq_SG_D_3_79fd4 : Inport  Port=2
  State_psi_q_SG_D_3_6a903 : Inport  Port=3
  State_theta_SG_D_3_fed8f : Inport  Port=4
  State_psi_1d_SG_D_3_f1d32 : Inport  Port=5
  State_psi_d_SG_D_3_cc5ad : Inport  Port=6
  State_psi_fd_SG_D_3_32316 : Inport  Port=7
  State_theta_SG_D_3_96b23 : Inport  Port=8
  Add_08435 : Sum
  Add_0e4e9 : Sum
  Add_2c759 : Sum
  Add_9cdd1 : Sum
  Add_a8142 : Sum
  Constant_-1_2427b : Constant  Value=-1
  Constant_-1_b33f2 : Constant  Value=-1
  Constant_-1_baa14 : Constant  Value=-1
  Constant_-1_db7da : Constant  Value=-1
  Constant_-1_df67d : Constant  Value=-1
  Constant_x_dd_55a1f : Constant  Value=x_dd
  Constant_x_dd_d809d : Constant  Value=x_dd
  Constant_x_dd_e64a8 : Constant  Value=x_dd
  Constant_x_ddd_07261 : Constant  Value=x_ddd
  Constant_x_ddd_62f2a : Constant  Value=x_ddd
  Constant_x_ddd_f2dd3 : Constant  Value=x_ddd
  Constant_x_l_3d32f : Constant  Value=x_l
  Constant_x_l_40019 : Constant  Value=x_l
  Constant_x_l_43e11 : Constant  Value=x_l
  Constant_x_l_982e9 : Constant  Value=x_l
  Constant_x_l_bc515 : Constant  Value=x_l
  Constant_x_l_fa61d : Constant  Value=x_l
  Constant_x_qd_4aa58 : Constant  Value=x_qd
  Constant_x_qd_6f554 : Constant  Value=x_qd
  Constant_x_qd_80ec9 : Constant  Value=x_qd
  Constant_x_qdd_039bf : Constant  Value=x_qdd
  Constant_x_qdd_11728 : Constant  Value=x_qdd
  Constant_x_qdd_cb4e5 : Constant  Value=x_qdd
  Divide_22075 : Product  Inputs=*/
  Divide_3e1c3 : Product  Inputs=*/
  Divide_53240 : Product  Inputs=*/
  Divide_b9e18 : Product  Inputs=*/
  Divide_d8290 : Product  Inputs=*/
  Divide_f1c67 : Product  Inputs=*/
  MathFunc_cos_6c1e4 : Trigonometry  Operator=cos
  MathFunc_sin_2aabc : Trigonometry
  Product_052da : Product
  Product_5bfc3 : Product
  Product_9a57c : Product
  Product_ab6bc : Product
  Product_c1409 : Product
  Product_c2cc9 : Product
  Product_c4573 : Product
  Product_ce554 : Product
  Product_d716c : Product
  Product_ddb54 : Product
  Product_e4dc9 : Product
  Subtract_0ae88 : Sum  Inputs=+-
  Subtract_1928c : Sum  Inputs=+-
  Subtract_25353 : Sum  Inputs=+-
  Subtract_32937 : Sum  Inputs=+-
  Subtract_37ddb : Sum  Inputs=+-
  Subtract_77d5b : Sum  Inputs=+-
  Subtract_978dc : Sum  Inputs=+-
  Subtract_a2099 : Sum  Inputs=+-
  Blockout_i_d_SG_D_3_fa4e4 : Outport
  wires:
  Constant_x_qd_80ec9/1 -> Subtract_37ddb/1
  Subtract_a2099/1 -> Blockout_i_d_SG_D_3_fa4e4/1
  Constant_-1_db7da/1 -> Product_9a57c/1
  Constant_x_l_43e11/1 -> Product_052da/2
  Constant_x_qdd_11728/1 -> Add_a8142/2
  Constant_x_qdd_039bf/1 -> Subtract_37ddb/2
  Constant_x_l_40019/1 -> Product_9a57c/2
  Divide_22075/1 -> Subtract_a2099/1
  Product_9a57c/1 -> Add_a8142/1
  Constant_x_ddd_07261/1 -> Subtract_1928c/2
  Constant_-1_baa14/1 -> Product_052da/1
  Constant_-1_2427b/1 -> Product_c1409/1
  Constant_x_l_bc515/1 -> Product_c1409/2
  State_psi_1d_SG_D_3_f1d32/1 -> Product_5bfc3/2
  State_psi_gq_SG_D_3_ef59b/1 -> Product_ce554/1
  Product_5bfc3/1 -> Product_ab6bc/1
  Add_a8142/1 -> Product_ce554/2
  Product_052da/1 -> Add_0e4e9/1
  Constant_x_qd_4aa58/1 -> Add_0e4e9/2
  State_psi_kq_SG_D_3_79fd4/1 -> Product_c2cc9/1
  Subtract_25353/1 -> Divide_d8290/2
  Subtract_37ddb/1 -> Product_c2cc9/2
  Product_c1409/1 -> Add_08435/1
  Constant_x_ddd_f2dd3/1 -> Subtract_0ae88/1
  Constant_x_qd_6f554/1 -> Add_08435/2
  Constant_-1_b33f2/1 -> Product_5bfc3/1
  Constant_x_dd_d809d/1 -> Subtract_1928c/1
  Product_ce554/1 -> Divide_b9e18/1
  Add_0e4e9/1 -> Divide_b9e18/2
  Product_c2cc9/1 -> Divide_53240/1
  Add_08435/1 -> Divide_53240/2
  Divide_d8290/1 -> Subtract_77d5b/2
  Subtract_1928c/1 -> Product_ab6bc/2
  State_theta_SG_D_3_fed8f/1 -> MathFunc_cos_6c1e4/1
  Constant_x_dd_55a1f/1 -> Subtract_978dc/1
  Product_c4573/1 -> Product_ddb54/1
  Constant_x_l_982e9/1 -> Subtract_978dc/2
  Add_2c759/1 -> Subtract_77d5b/1
  Constant_x_l_fa61d/1 -> Subtract_0ae88/2
  State_theta_SG_D_3_96b23/1 -> MathFunc_sin_2aabc/1
  Divide_b9e18/1 -> Subtract_32937/1
  Add_9cdd1/1 -> Product_c4573/2
  Divide_53240/1 -> Subtract_32937/2
  Product_ab6bc/1 -> Divide_f1c67/1
  Subtract_978dc/1 -> Divide_f1c67/2
  State_psi_fd_SG_D_3_32316/1 -> Product_e4dc9/1
  Divide_3e1c3/1 -> Subtract_a2099/2
  Subtract_0ae88/1 -> Product_e4dc9/2
  Constant_x_dd_e64a8/1 -> Subtract_25353/1
  Subtract_32937/1 -> Add_9cdd1/1
  Constant_x_l_3d32f/1 -> Subtract_25353/2
  Constant_-1_df67d/1 -> Product_c4573/1
  State_psi_q_SG_D_3_6a903/1 -> Add_9cdd1/2
  Divide_f1c67/1 -> Add_2c759/1
  State_psi_d_SG_D_3_cc5ad/1 -> Add_2c759/2
  Product_e4dc9/1 -> Divide_d8290/1
  MathFunc_cos_6c1e4/1 -> Product_ddb54/2
  MathFunc_sin_2aabc/1 -> Product_d716c/2
  Subtract_77d5b/1 -> Product_d716c/1
  Product_ddb54/1 -> Divide_22075/1
  Constant_x_qdd_cb4e5/1 -> Divide_22075/2
  Product_d716c/1 -> Divide_3e1c3/1
  Constant_x_ddd_62f2a/1 -> Divide_3e1c3/2
